simulink model "anti_windup_deadzone_discrete_spring16"  (R2015b)
settings: Solver=ode45  StartTime=0.0  StopTime=40.0  RelTol=1e-3
values from neighbouring files (symbols this model uses):
  h = 0.14    [L9.m]    (also in anti_windup_analysis.m = 0.0918594343155; anti_windup_spring16.m = 0.1)
  K = 0.6*Ku    (= 1.548)    [anti_windup_spring16.m]    (also in tank_PID_tuning.m = 39.66)
  N = 15    [anti_windup_analysis.m]    (also in anti_windup_spring16.m; tank_PID_tuning.m = 20)
  Td = Tu/8    (= 0.384999099705)    [PID_parameters_Carr_1986_example.m]    (also in anti_windup_analysis.m = 0.514358797205; anti_windup_spring16.m = 0.18125; tank_PID_tuning.m = 4.53125)
  Ti = Tu/2    (= 1.53999639882)    [PID_parameters_Carr_1986_example.m]    (also in anti_windup_analysis.m = 3.07999279764; anti_windup_spring16.m = 0.725; tank_PID_tuning.m = 18.125)
  Tt = 2*Ti    (= 6.15998559527)    [anti_windup_analysis.m]    (also in anti_windup_spring16.m = 0.3625)
  uHigh = 0.2    [anti_windup_analysis.m]    (also in anti_windup_spring16.m = 0.7)
  uLow = -0.2    [anti_windup_analysis.m]    (also in anti_windup_spring16.m = -0.7)
undefined symbols (not defined in the file or in its folder): A1, A2, B1, B2
settings Model: Creator=kjartan  LastModifiedBy=kjartan
settings DataIOCC: SaveFormat=Array
settings DebuggingCC: SolverPrmCheckMsg=warning
settings HardwareCC: ProdBitPerPointer=32  ProdLargestAtomicFloat=None  ProdIntDivRoundTo=Undefined  ProdEndianess=Unspecified  ProdWordSize=32  ProdHWDeviceType=32-bit Generic
settings GRTTargetCC: GeneratePreprocessorConditionals=Disable all
settings ConfigComp: CovModelRefEnable=Off  CovSFcnEnable=off

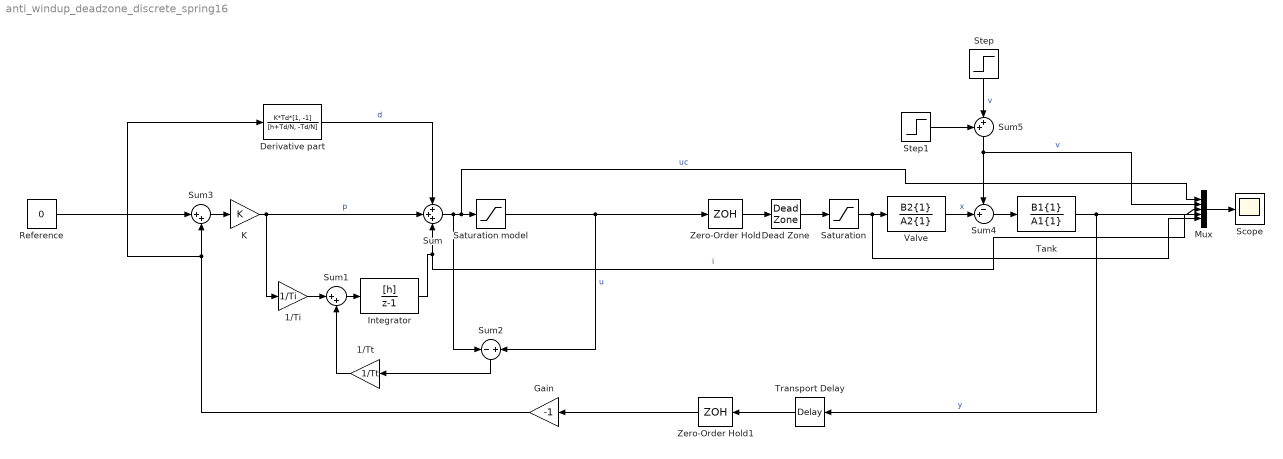
== system anti_windup_deadzone_discrete_spring16 ==
  1/Ti : Gain  Gain=1/Ti
  1/Tt : Gain  Gain=1/Tt
  Dead Zone : DeadZone  LowerValue=-0.2  UpperValue=0.2  SaturateOnIntegerOverflow=on
  Derivative part : DiscreteFilter  Numerator=K*Td*[1, -1]  Denominator=[h+Td/N, -Td/N]  SampleTime=h
  Gain : Gain  Gain=-1
  Integrator : DiscreteTransferFcn  Numerator=[h]  Denominator=[1 -1]  SampleTime=h
  K : Gain  Gain=K
  Mux : Mux  Inputs=5
  Reference : Constant  Value=0
  Saturation : Saturate  UpperLimit=uHigh  LowerLimit=uLow
  Saturation model : Saturate  UpperLimit=uHigh  LowerLimit=uLow
  Scope : Scope
  Step : Step  Time=5  SampleTime=0
  Step1 : Step  Time=20  After=-1  SampleTime=0
  Sum : Sum  Inputs=+++
  Sum1 : Sum  Inputs=|++
  Sum2 : Sum  Inputs=-|+
  Sum3 : Sum  Inputs=|++
  Sum4 : Sum  Inputs=-+|
  Sum5 : Sum  Inputs=++|
  Tank : TransferFcn  Numerator=B1{1}  Denominator=A1{1}
  Transport Delay : TransportDelay  DelayTime=0.1
  Valve : TransferFcn  Numerator=B2{1}  Denominator=A2{1}
  Zero-Order Hold : ZeroOrderHold  SampleTime=h
  Zero-Order Hold1 : ZeroOrderHold  SampleTime=h
  wires:
  Saturation model/1 -> Zero-Order Hold/1, Sum2/2  "u"
  Sum/1 -> Mux/1, Saturation model/1, Sum2/1  "uc"
  Derivative part/1 -> Sum/1  "d"
  K/1 -> 1/Ti/1, Sum/2  "p"
  1/Ti/1 -> Sum1/1
  Sum1/1 -> Integrator/1
  Integrator/1 -> Sum/3, Mux/4  "i"
  Sum2/1 -> 1/Tt/1
  1/Tt/1 -> Sum1/2
  Reference/1 -> Sum3/1
  Sum3/1 -> K/1
  Mux/1 -> Scope/1
  Gain/1 -> Derivative part/1, Sum3/2
  Zero-Order Hold1/1 -> Gain/1
  Saturation/1 -> Mux/5, Valve/1
  Sum4/1 -> Tank/1
  Tank/1 -> Transport Delay/1, Mux/3  "y"
  Transport Delay/1 -> Zero-Order Hold1/1
  Valve/1 -> Sum4/2  "x"
  Sum5/1 -> Mux/2, Sum4/1  "v"
  Step/1 -> Sum5/2  "v"
  Step1/1 -> Sum5/1
  Zero-Order Hold/1 -> Dead Zone/1
  Dead Zone/1 -> Saturation/1
